simulink model "Attitude_Control"  (R2018b)
settings: Solver=VariableStepAuto  StartTime=0.0  StopTime=500.0  RelTol=1e-3  EnableMultiTasking=on
values from neighbouring files (symbols this model uses):
  kd = .01    (= 0.01)    [Rigid_Body_Sim.m]    (also in Sim_init.m = 0.068)
  kp = 1    [Rigid_Body_Sim.m]    (also in Sim_init.m = wn.^2)
  qd = [ 0.9973 ... (first row only)    [Sim_init.m]
libraries: aerolibutil x2, Satellite_Dynamics x1
settings Model: Creator=devantormey  LastModifiedBy=devantormey
settings OptimizationCC: LifeSpan=inf
settings DebuggingCC: SFUnexpectedBacktrackingDiag=warning  SFNoUnconditionalDefaultTransitionDiag=warning
settings SFSimCC: SimUseLocalCustomCode=off
settings RTWCC: RTWUseLocalCustomCode=off
settings CodeAppCC: StateflowObjectComments=on
settings GRTTargetCC: TargetLangStandard=C89/C90 (ANSI)  GeneratePreprocessorConditionals=Disable all
settings ConfigComp: CovMetricSettings=dw  CovHtmlReporting=on  CovSaveCumulativeToWorkspaceVar=on  CovSaveSingleToWorkspaceVar=on  CovExternalEMLEnable=off

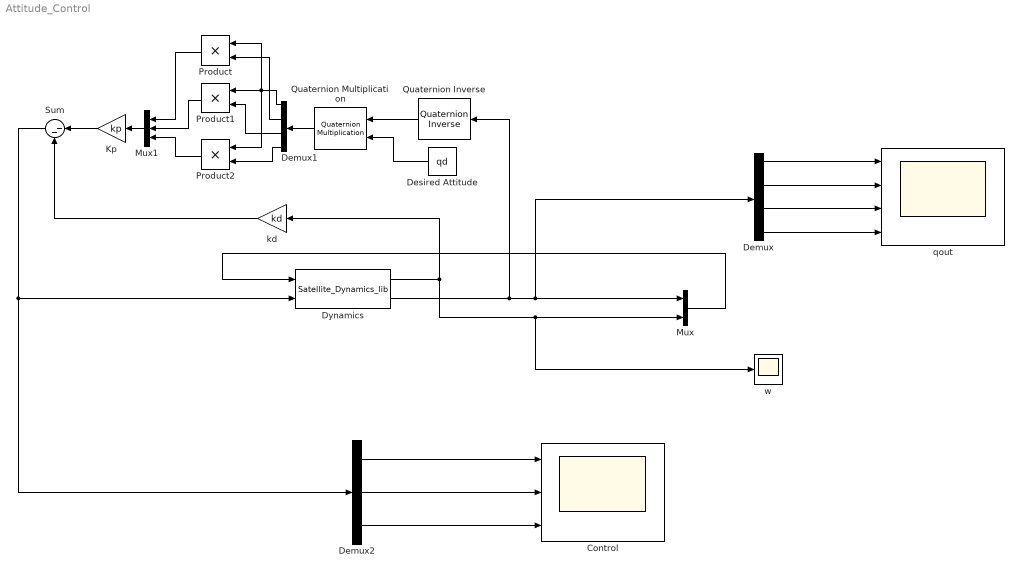
== system Attitude_Control ==
  Control : Scope  NumInputPorts=3
  Demux : Demux
  Demux1 : Demux
  Demux2 : Demux  Outputs=3
  Desired Attitude : Constant  Value=qd
  "Dynamics " : Satellite_Dynamics/Satellite_Dynamics_lib  SystemSampleTime=-1
  Kp : Gain  Gain=kp
  Mux : Mux  Inputs=2
  Mux1 : Mux  Inputs=3
  Product : Product
  Product1 : Product
  Product2 : Product
  Quaternion Inverse : aerolibutil/Quaternion Inverse
      settings: SourceProductName=Aerospace Blockset
  Quaternion Multiplication : aerolibutil/Quaternion Multiplication
  Sum : Sum  Inputs=|--
  kd : Gain  Gain=kd
  qout : Scope  NumInputPorts=4
  w : Scope
  wires:
  "Dynamics "/2 -> Quaternion Inverse/1, Demux/1, Mux/1
  Mux/1 -> "Dynamics "/1
  Demux/1 -> qout/1
  Demux/2 -> qout/2
  Demux/3 -> qout/3
  Demux/4 -> qout/4
  "Dynamics "/1 -> kd/1, w/1, Mux/2
  kd/1 -> Sum/2
  Sum/1 -> "Dynamics "/2, Demux2/1
  Demux2/2 -> Control/2
  Demux2/1 -> Control/1
  Demux2/3 -> Control/3
  Kp/1 -> Sum/1
  Quaternion Inverse/1 -> Quaternion Multiplication/1
  Desired Attitude/1 -> Quaternion Multiplication/2
  Quaternion Multiplication/1 -> Demux1/1
  Demux1/1 -> Product2/1, Product/1, Product1/1
  Demux1/2 -> Product/2
  Demux1/3 -> Product1/2
  Demux1/4 -> Product2/2
  Mux1/1 -> Kp/1
  Product/1 -> Mux1/1
  Product1/1 -> Mux1/2
  Product2/1 -> Mux1/3
